simulink model "PMSM_MRAS"  (R2014b)
settings: Solver=ode23tb  StartTime=0.0  StopTime=0.4  FixedStep=5e-5  RelTol=1e-3
InitFcn:
  | L=8.5e-3;
  | R=2.875;
  | flux=0.175;
libraries: powerlib_extras x4, powerlib x4, simulink x1
settings Model: Creator=Paladin611  LastModifiedBy=Lei
settings DataIOCC: LimitDataPoints=off  SignalLoggingSaveFormat=ModelDataLogs
settings OptimizationCC: ExpressionDepthLimit=2147483647  InitFltsAndDblsToZero=on  EfficientMapNaN2IntZero=off
settings DebuggingCC: SaveWithParameterizedLinksMsg=none  UnderspecifiedInitializationDetection=Classic  MergeDetectMultiDrivingBlocksExec=none  SignalResolutionControl=TryResolveAllWithWarning  MultiTaskDSMMsg=warning  MultiTaskCondExecSysMsg=none  FcnCallInpInsideContextMsg=UseLocalSettings  StateNameClashWarn=warning
settings HardwareCC: TargetEndianess=LittleEndian  TargetHWDeviceType=MATLAB Host  ProdEqTarget=off
settings CodeAppCC: MaxIdLength=128
settings GRTTargetCC: CombineOutputUpdateFcns=off  GRTInterface=on

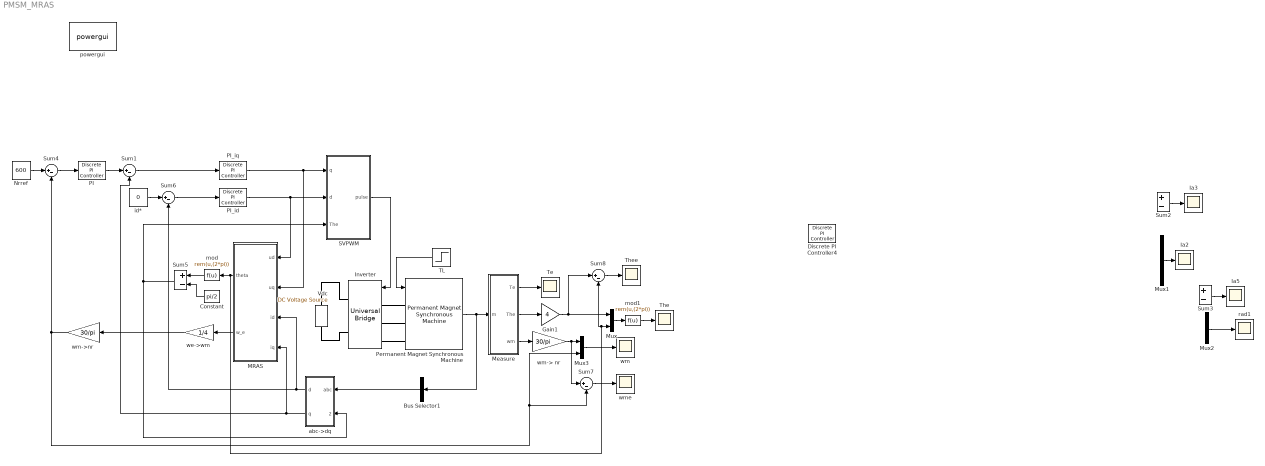
== system PMSM_MRAS ==
  Bus Selector1 : BusSelector  OutputSignals=Stator current is_a (A),Stator current is_b (A),Stator current is_c (A)  OutputAsBus=on
  Constant : Constant  Value=pi/2
  Discrete PI Controller4 : powerlib_extras/Discrete  Control Blocks/Discrete PI Controller  Kp=1*15  Ki=1000*4  Par_Limits=[1000 -1000]  Init=0  Ts=10e-6
  Gain1 : Gain  Gain=4
  Ia2 : Scope
      settings: TimeRange=0.1  YMin=-2  YMax=6.5  SaveName=ScopeData6
  Ia3 : Scope
      settings: TimeRange=0.1167052469135803  YMin=-6.5  YMax=2  SaveName=ScopeData7
  Ia5 : Scope
      settings: TimeRange=0.5  YMin=-100  YMax=150  SaveName=ScopeData11
  Inverter : powerlib/Power Electronics/Universal Bridge  Arms=3  SnubberResistance=1e5  SnubberCapacitance=inf  Device=IGBT / Diodes  Ron=1e-3  Lon=0  ForwardVoltages="[  0  0  ]"  ForwardVoltage=0  GTOparameters=[ 10e-6 , 20e-6 ]  IGBTparameters=[ 1e-6 , 2e-6 ]  Measurements=None  Measurements_2=None  converterType=Rectifier
  MRAS : Subsystem
  Measure : Subsystem
  Mux{,1..3} (4 alike) : Mux  Inputs=2
  Nrref : Constant  Value=600
  PI : powerlib_extras/Discrete  Control Blocks/Discrete PI Controller  Kp=0.068  Ki=17.1  Par_Limits=[100 -100]  Init=0  Ts=10e-6
  PI_id : powerlib_extras/Discrete  Control Blocks/Discrete PI Controller  Kp=L*2000  Ki=R*2000  Par_Limits=[300 -300]  Init=0  Ts=10e-6
  PI_iq : powerlib_extras/Discrete  Control Blocks/Discrete PI Controller  Kp=L*2000  Ki=R*2000  Par_Limits=[300 -300]  Init=0  Ts=10e-6
  Permanent Magnet Synchronous Machine : powerlib/Machines/Permanent Magnet Synchronous Machine  NbPhases=3  FluxDistribution=Sinusoidal  RotorType=Salient-pole  MechanicalLoad=Torque Tm  PresetModel=No  ShowDetailedParameters=on  MeasurementBus=off  Resistance=2.875  Inductance=8.5e-3  dqInductances=[8.5e-3 8.5e-3]  La=0.00085  MachineConstant=Flux linkage established by magnets (V.s)  Flux=0.175  VoltageCst=126.966  TorqueCst=1.05  Flat=120  Mechanical=[4.8e-6,0,4,0]  PolePairs=4  InitialConditions=[0,0, 0,0]  InitialConditions5ph=[0 0 0 0 0 0]  TsPowergui=0  TsBlock=-1  RefAngle=Aligned with phase A axis (original Park)
  SVPWM : Subsystem
  Sum{1,4,6..8} (5 alike) : Sum  Inputs=|+-
  Sum2 : Sum  Inputs=+-
  Sum3 : Sum  Inputs=+-
  Sum5 : Sum  Inputs=+-
  TL : Step  Time=0.3  After=0  SampleTime=0
  Te : Scope
      settings: TimeRange=0.01478751540608518  YMin=-7.5e-19  YMax=7.5e-19  SaveName=ScopeData10
  The : Scope
      settings: YMin=4.8  YMax=6.2  SaveName=The
  Thee : Scope
      settings: YMin=-0.4  YMax=0.05  SaveName=The1
  Vdc : powerlib/Electrical Sources/DC Voltage Source  Amplitude=311  Measurements=None
  abc->dq : Subsystem
  id* : Constant  Value=0
  mod : Fcn  Expr=rem(u,(2*pi))
  mod1 : Fcn  Expr=rem(u,(2*pi))
  powergui : powerlib/powergui  Priority=1  SimulationMode=Continuous  SolverType=Tustin  SampleTime=1e-6  frequency=60  SPID=off  DisableSnubberDevices=off  DisableRonSwitches=off  DisableVfSwitches=off  SwTol=0  DisplayEquations=off  Interpol=off  methode=off  Ts=0  frequencyindice=0  Pbase=100e6  ErrMax=1e-4  Iterations=50  UnitsV=kV  UnitsW=MW  FunctionMessages=off  echomessages=off  HookPort=off  EnableUseOfTLC=off  x0status=blocks  RestoreLinks=warning  ResistiveCurrentMeasurement=off  Frange=[0:2:500]  Ylog=off  Xlog=on  ShowGrid=off  save=off  variable=ZData  structure=0  ZoomFFT=off  StartTime=0.0  cycles=1  DisplayStyle=1  fundamental=60  FreqAxis=off  MaxFrequency=1000  frequencyindicesteady=1  RmsSteady=1  display=off
  rad1 : Scope
      settings: TimeRange=0.1  YMin=20  YMax=110  SaveName=ScopeData9
  we->wm : Gain  Gain=1/4
  wm : Scope
      settings: TimeRange=0.4  YMin=-200  YMax=1200  SaveName=wm
  wm-> nr : Gain  Gain=30/pi
  wm->nr : Gain  Gain=30/pi
  wme : Scope
      settings: TimeRange=0.4  YMin=-400  YMax=300  SaveName=wm1
  wires:
  Permanent Magnet Synchronous Machine/1 -> Measure/1(m), Bus Selector1/1
  Sum4/1 -> PI/1
  Sum1/1 -> PI_iq/1
  Sum6/1 -> PI_id/1
  Nrref/1 -> Sum4/1
  PI/1 -> Sum1/1
  Constant/1 -> Sum5/2
  ? -> Sum3/2, Mux2/2  "<Rotor speed wm (rad/s)>"
  ? -> Sum3/1, Mux2/1
  Mux1/1 -> Ia2/1
  Mux2/1 -> rad1/1
  Sum3/1 -> Ia5/1
  Sum2/1 -> Ia3/1
  ? -> Sum2/1
  ? -> Sum2/2
  ? -> Mux1/1
  ? -> Mux1/2
  id*/1 -> Sum6/1
  SVPWM/1(pulse) -> Inverter/1
  abc->dq/1(d) -> MRAS/3(id), Sum6/2
  abc->dq/2(q) -> Sum1/2, MRAS/4(iq)
  MRAS/2(w_e) -> we->wm/1
  we->wm/1 -> wm->nr/1
  Sum5/1 -> abc->dq/2(theta), SVPWM/3(The)
  PI_iq/1 -> MRAS/2(uq), SVPWM/1(q)
  PI_id/1 -> MRAS/1(ud), SVPWM/2(d)
  Measure/1(Te) -> Te/1
  Measure/2(The) -> Gain1/1
  Bus Selector1/1 -> abc->dq/1(abc)
  mod/1 -> Sum5/1
  Measure/3(wm) -> wm-> nr/1
  Mux3/1 -> wm/1
  wm->nr/1 -> Sum7/2, Mux3/2, Sum4/2
  wm-> nr/1 -> Sum7/1, Mux3/1
  Sum7/1 -> wme/1
  Sum8/1 -> Thee/1
  TL/1 -> Permanent Magnet Synchronous Machine/1
  Mux/1 -> mod1/1
  Gain1/1 -> Mux/1, Sum8/1
  MRAS/1(theta) -> Sum8/2, Mux/2, mod/1
  mod1/1 -> The/1
  connections:
  Vdc/LConn1 -- Inverter/RConn2
  Permanent Magnet Synchronous Machine/LConn1 -- Inverter/LConn1
  Permanent Magnet Synchronous Machine/LConn2 -- Inverter/LConn2
  Permanent Magnet Synchronous Machine/LConn3 -- Inverter/LConn3
  Vdc/RConn1 -- Inverter/RConn1

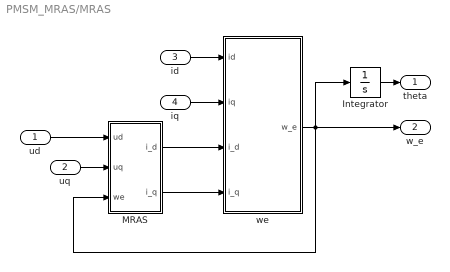
== system PMSM_MRAS/MRAS ==
  ud : Inport
  uq : Inport  Port=2
  id : Inport  Port=3
  iq : Inport  Port=4
  Integrator : Integrator
  MRAS : Subsystem
  we : Subsystem
  theta : Outport
  w_e : Outport  Port=2
  wires:
  ud/1 -> MRAS/1(ud)
  iq/1 -> we/2(iq)
  we/1(w_e) -> MRAS/3(we), w_e/1, Integrator/1
  uq/1 -> MRAS/2(uq)
  Integrator/1 -> theta/1
  MRAS/2(i_q) -> we/4(i_q)
  id/1 -> we/1(id)
  MRAS/1(i_d) -> we/3(i_d)

== system PMSM_MRAS/Measure ==
  m : Inport
  Bus Selector : BusSelector  OutputSignals=Electromagnetic torque Te (N*m),Rotor angle thetam (rad),Rotor speed wm (rad/s)
  Te : Outport
  The : Outport  Port=2
  wm : Outport  Port=3
  wires:
  Bus Selector/1 -> Te/1  "<Electromagnetic torque Te (N*m)>"
  Bus Selector/3 -> wm/1  "<Rotor speed wm (rad/s)>"
  Bus Selector/2 -> The/1  "<Rotor angle thetam (rad)>"
  m/1 -> Bus Selector/1

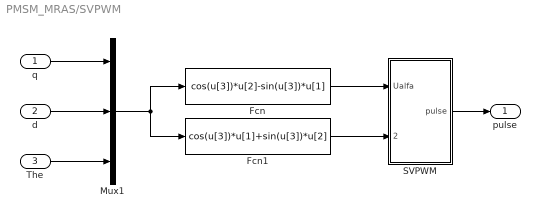
== system PMSM_MRAS/SVPWM ==
  q : Inport
  d : Inport  Port=2
  The : Inport  Port=3
  Fcn : Fcn  Expr=cos(u[3])*u[2]-sin(u[3])*u[1]
  Fcn1 : Fcn  Expr=cos(u[3])*u[1]+sin(u[3])*u[2]
  Mux1 : Mux  Inputs=3
  SVPWM : Subsystem  Tag=SVPWM  mask{F=10, Vdc=311}
      mask prompts: F "Chopping　Frequency(KHz)"; Vdc "DC Voltage(V)"
  pulse : Outport
  wires:
  The/1 -> Mux1/3
  Mux1/1 -> Fcn1/1, Fcn/1
  d/1 -> Mux1/2
  q/1 -> Mux1/1
  Fcn/1 -> SVPWM/1(Ualfa)
  Fcn1/1 -> SVPWM/2(Ubeta)
  SVPWM/1(pulse) -> pulse/1

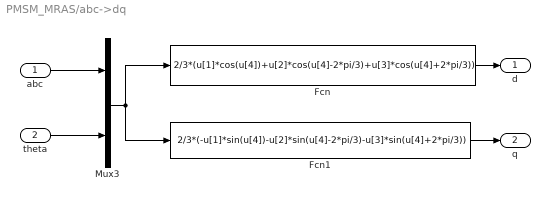
== system PMSM_MRAS/abc->dq ==
  abc : Inport
  theta : Inport  Port=2
  Fcn : Fcn  Expr=2/3*(u[1]*cos(u[4])+u[2]*cos(u[4]-2*pi/3)+u[3]*cos(u[4]+2*pi/3))
  Fcn1 : Fcn  Expr=2/3*(-u[1]*sin(u[4])-u[2]*sin(u[4]-2*pi/3)-u[3]*sin(u[4]+2*pi/3))
  Mux3 : Mux  Inputs=2
  d : Outport
  q : Outport  Port=2
  wires:
  Mux3/1 -> Fcn1/1, Fcn/1
  theta/1 -> Mux3/2
  Fcn/1 -> d/1
  Fcn1/1 -> q/1
  abc/1 -> Mux3/1

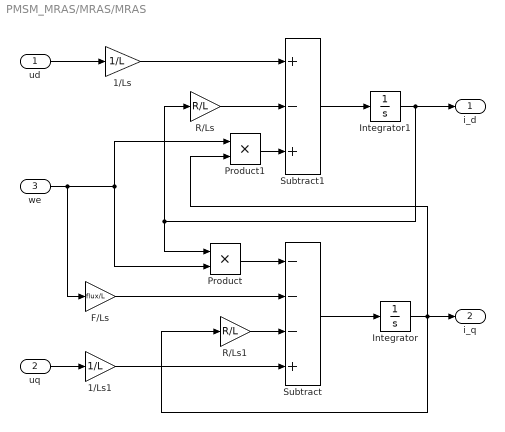
== system PMSM_MRAS/MRAS/MRAS ==
  ud : Inport
  uq : Inport  Port=2
  we : Inport  Port=3
  1/Ls : Gain  Gain=1/L
  1/Ls1 : Gain  Gain=1/L
  F/Ls : Gain  Gain=flux/L
  Integrator : Integrator
  Integrator1 : Integrator
  Product : Product  RndMeth=Zero
  Product1 : Product  RndMeth=Zero
  R/Ls : Gain  Gain=R/L
  R/Ls1 : Gain  Gain=R/L
  Subtract : Sum  Inputs=---+
  Subtract1 : Sum  Inputs=+-+
  i_d : Outport
  i_q : Outport  Port=2
  wires:
  1/Ls1/1 -> Subtract/4
  Subtract/1 -> Integrator/1
  Subtract1/1 -> Integrator1/1
  1/Ls/1 -> Subtract1/1
  Product1/1 -> Subtract1/3
  R/Ls/1 -> Subtract1/2
  Product/1 -> Subtract/1
  R/Ls1/1 -> Subtract/3
  uq/1 -> 1/Ls1/1
  we/1 -> F/Ls/1, Product/2, Product1/1
  F/Ls/1 -> Subtract/2
  Integrator1/1 -> R/Ls/1, Product/1, i_d/1
  ud/1 -> 1/Ls/1
  Integrator/1 -> R/Ls1/1, i_q/1, Product1/2

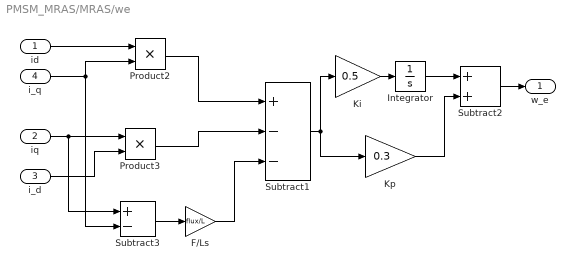
== system PMSM_MRAS/MRAS/we ==
  id : Inport
  iq : Inport  Port=2
  i_d : Inport  Port=3
  i_q : Inport  Port=4
  F/Ls : Gain  Gain=flux/L
  Integrator : Integrator
  Ki : Gain  Gain=0.5
  Kp : Gain  Gain=0.3
  Product2 : Product  RndMeth=Zero
  Product3 : Product  RndMeth=Zero
  Subtract1 : Sum  Inputs=+--
  Subtract2 : Sum
  Subtract3 : Sum  Inputs=+-
  w_e : Outport
  wires:
  id/1 -> Product2/1
  i_q/1 -> Subtract3/2, Product2/2
  iq/1 -> Subtract3/1, Product3/1
  i_d/1 -> Product3/2
  Subtract3/1 -> F/Ls/1
  F/Ls/1 -> Subtract1/3
  Subtract1/1 -> Ki/1, Kp/1
  Ki/1 -> Integrator/1
  Integrator/1 -> Subtract2/1
  Kp/1 -> Subtract2/2
  Product2/1 -> Subtract1/1
  Product3/1 -> Subtract1/2
  Subtract2/1 -> w_e/1

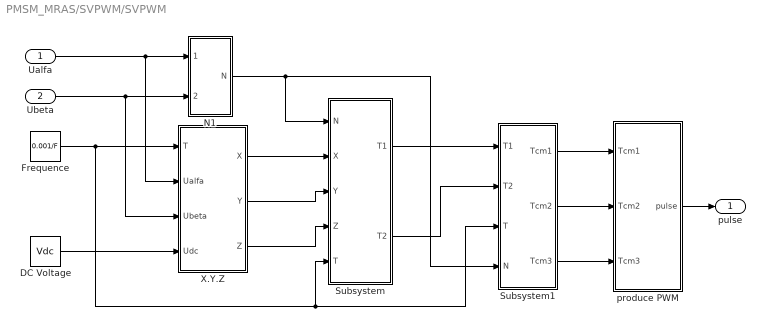
== system PMSM_MRAS/SVPWM/SVPWM ==
  Ualfa : Inport
  Ubeta : Inport  Port=2
  DC Voltage : Constant  Value=Vdc
  Frequence : Constant  Value=0.001/F
  N1 : Subsystem
  Subsystem : Subsystem
  Subsystem1 : Subsystem
  X.Y.Z : Subsystem
  produce PWM : Subsystem
  pulse : Outport
  wires:
  Ubeta/1 -> X.Y.Z/3(Ubeta), N1/2(Ubeta)
  Subsystem/2(T2) -> Subsystem1/2(T2)
  Subsystem/1(T1) -> Subsystem1/1(T1)
  Ualfa/1 -> N1/1(Ualfa), X.Y.Z/2(Ualfa)
  Subsystem1/3(Tcm3) -> produce PWM/3(Tcm3)
  Subsystem1/2(Tcm2) -> produce PWM/2(Tcm2)
  Subsystem1/1(Tcm1) -> produce PWM/1(Tcm1)
  X.Y.Z/3(Z) -> Subsystem/4(Z)
  X.Y.Z/2(Y) -> Subsystem/3(Y)
  X.Y.Z/1(X) -> Subsystem/2(X)
  N1/1(N) -> Subsystem1/4(N), Subsystem/1(N)
  DC Voltage/1 -> X.Y.Z/4(Udc)
  Frequence/1 -> Subsystem/5(T), Subsystem1/3(T), X.Y.Z/1(T)
  produce PWM/1(pulse) -> pulse/1

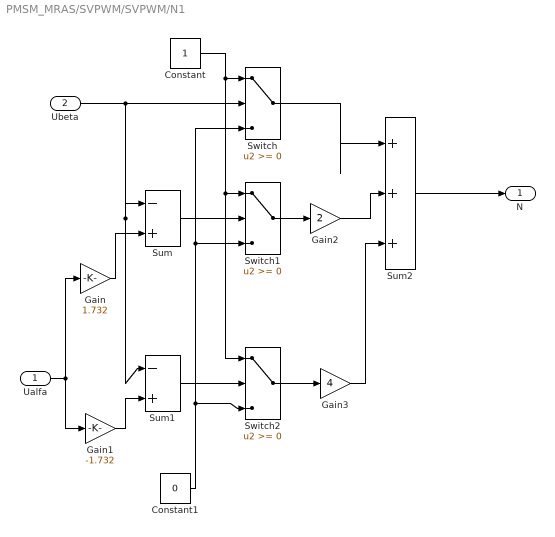
== system PMSM_MRAS/SVPWM/SVPWM/N1 ==
  Ualfa : Inport
  Ubeta : Inport  Port=2
  Constant : Constant
  Constant1 : Constant  Value=0
  Gain : Gain  Gain=1.732
  Gain1 : Gain  Gain=-1.732
  Gain2 : Gain  Gain=2
  Gain3 : Gain  Gain=4
  Sum : Sum  Inputs=|-+
  Sum1 : Sum  Inputs=|-+
  Sum2 : Sum  Inputs=|+++
  Switch : Switch
  Switch1 : Switch
  Switch2 : Switch
  N : Outport
  wires:
  Sum2/1 -> N/1
  Gain3/1 -> Sum2/3
  Switch/1 -> Sum2/1
  Gain2/1 -> Sum2/2
  Switch2/1 -> Gain3/1
  Switch1/1 -> Gain2/1
  Constant1/1 -> Switch2/3, Switch1/3, Switch/3
  Gain1/1 -> Sum1/2
  Sum1/1 -> Switch2/2
  Sum/1 -> Switch1/2
  Gain/1 -> Sum/2
  Ualfa/1 -> Gain/1, Gain1/1
  Constant/1 -> Switch1/1, Switch2/1, Switch/1
  Ubeta/1 -> Sum1/1, Sum/1, Switch/2

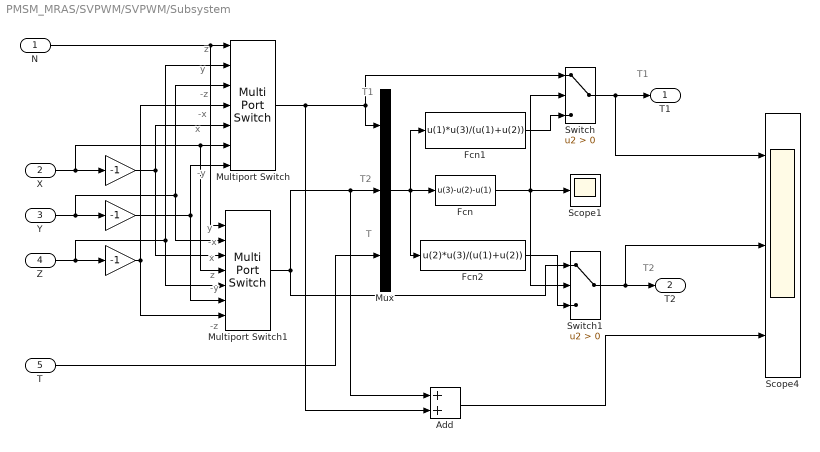
== system PMSM_MRAS/SVPWM/SVPWM/Subsystem ==
  note: T2
  note: T1
  note: T
  note: T2
  note: T1
  note: -z
  note: -y
  note: z
  note: x
  note: -x
  note: y
  note: -y
  note: x
  note: -x
  note: -z
  note: y
  note: z
  N : Inport
  X : Inport  Port=2
  Y : Inport  Port=3
  Z : Inport  Port=4
  T : Inport  Port=5
  " " : Gain  Gain=-1
  "  " : Gain  Gain=-1
  "    " : Gain  Gain=-1
  Add : Sum
  Fcn : Fcn  Expr=u(3)-u(2)-u(1)
  Fcn1 : Fcn  Expr=u(1)*u(3)/(u(1)+u(2))
  Fcn2 : Fcn  Expr=u(2)*u(3)/(u(1)+u(2))
  Multiport Switch : MultiPortSwitch  Inputs=6  DiagnosticForDefault=None
  Multiport Switch1 : MultiPortSwitch  Inputs=6  DiagnosticForDefault=None
  Mux : Mux  Inputs=3
  Scope1 : Scope
      settings: YMin=2  YMax=6  SaveName=ScopeData16
  Scope4 : Scope  NumInputPorts=3
      settings: TimeRange=0.5  YMin=-5e-05~-5e-05~0  YMax=9.999999999999999e-05~9.999999999999999e-05~0.008  SaveName=ScopeData4
  Switch : Switch  Criteria=u2 > Threshold
  Switch1 : Switch  Criteria=u2 > Threshold
  T1 : Outport
  T2 : Outport  Port=2
  wires:
  Add/1 -> Scope4/3
  Switch1/1 -> Scope4/2, T2/1
  Switch/1 -> Scope4/1, T1/1
  Fcn2/1 -> Switch1/3
  Fcn1/1 -> Switch/3
  Mux/1 -> Fcn2/1, Fcn1/1, Fcn/1
  T/1 -> Mux/3
  Multiport Switch/1 -> Add/2, Switch/1, Mux/1
  " "/1 -> Multiport Switch1/3, Multiport Switch/5
  "  "/1 -> Multiport Switch1/6, Multiport Switch/7
  "    "/1 -> Multiport Switch/4, Multiport Switch1/7
  Z/1 -> "    "/1, Multiport Switch/2, Multiport Switch1/5
  Y/1 -> "  "/1, Multiport Switch/3, Multiport Switch1/2
  X/1 -> " "/1, Multiport Switch/6, Multiport Switch1/4
  N/1 -> Multiport Switch/1, Multiport Switch1/1
  Fcn/1 -> Scope1/1, Switch1/2, Switch/2
  Multiport Switch1/1 -> Add/1, Mux/2, Switch1/1

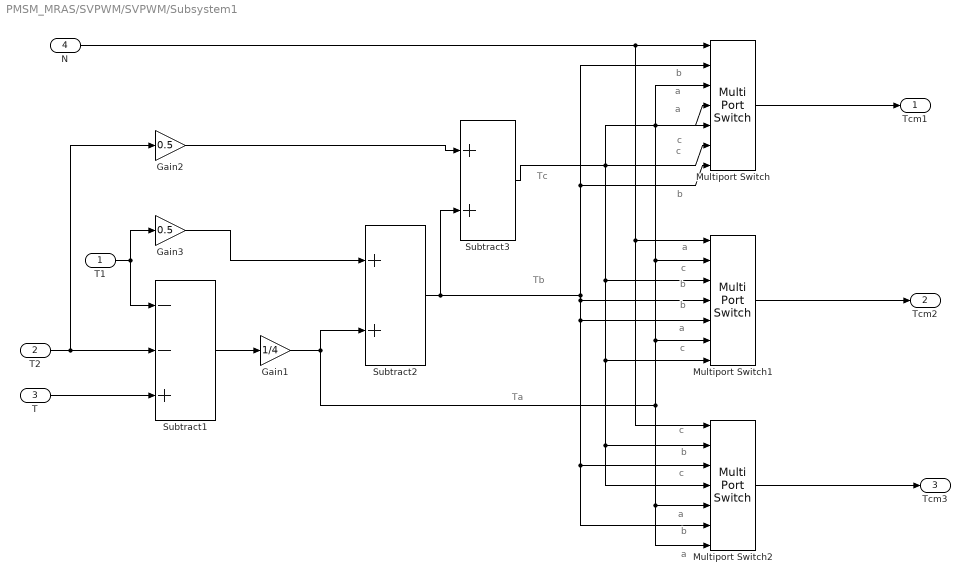
== system PMSM_MRAS/SVPWM/SVPWM/Subsystem1 ==
  note: a
  note: b
  note: a
  note: c
  note: b
  note: c
  note: c
  note: a
  note: b
  note: b
  note: c
  note: a
  note: b
  note: c
  note: c
  note: a
  note: a
  note: b
  note: Tc
  note: Tb
  note: Ta
  T1 : Inport
  T2 : Inport  Port=2
  T : Inport  Port=3
  N : Inport  Port=4
  Gain1 : Gain  Gain=1/4
  Gain2 : Gain  Gain=0.5
  Gain3 : Gain  Gain=0.5
  Multiport Switch : MultiPortSwitch  Inputs=6  DiagnosticForDefault=None
  Multiport Switch1 : MultiPortSwitch  Inputs=6  DiagnosticForDefault=None
  Multiport Switch2 : MultiPortSwitch  Inputs=6  DiagnosticForDefault=None
  Subtract1 : Sum  Inputs=--+
  Subtract2 : Sum
  Subtract3 : Sum
  Tcm1 : Outport
  Tcm2 : Outport  Port=2
  Tcm3 : Outport  Port=3
  wires:
  Subtract3/1 -> Multiport Switch2/4, Multiport Switch2/2, Multiport Switch1/7, Multiport Switch1/3, Multiport Switch/6, Multiport Switch/5
  N/1 -> Multiport Switch1/1, Multiport Switch2/1, Multiport Switch/1
  Gain2/1 -> Subtract3/1
  Subtract2/1 -> Multiport Switch2/6, Multiport Switch2/3, Multiport Switch1/5, Multiport Switch1/4, Multiport Switch/7, Multiport Switch/2, Subtract3/2
  Gain1/1 -> Subtract2/2, Multiport Switch1/6, Multiport Switch1/2, Multiport Switch/4, Multiport Switch/3, Multiport Switch2/7, Multiport Switch2/5
  Subtract1/1 -> Gain1/1
  Gain3/1 -> Subtract2/1
  T1/1 -> Subtract1/1, Gain3/1
  T/1 -> Subtract1/3
  T2/1 -> Subtract1/2, Gain2/1
  Multiport Switch/1 -> Tcm1/1
  Multiport Switch1/1 -> Tcm2/1
  Multiport Switch2/1 -> Tcm3/1

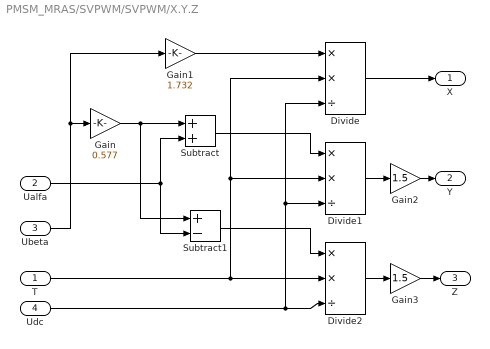
== system PMSM_MRAS/SVPWM/SVPWM/X.Y.Z ==
  T : Inport
  Ualfa : Inport  Port=2
  Ubeta : Inport  Port=3
  Udc : Inport  Port=4
  Divide : Product  Inputs=**/
  Divide1 : Product  Inputs=**/
  Divide2 : Product  Inputs=**/
  Gain : Gain  Gain=0.577
  Gain1 : Gain  Gain=1.732
  Gain2 : Gain  Gain=1.5
  Gain3 : Gain  Gain=1.5
  Subtract : Sum
  Subtract1 : Sum  Inputs=+-
  X : Outport
  Y : Outport  Port=2
  Z : Outport  Port=3
  wires:
  Ubeta/1 -> Gain/1, Gain1/1
  Gain3/1 -> Z/1
  Gain2/1 -> Y/1
  Divide2/1 -> Gain3/1
  Divide1/1 -> Gain2/1
  Divide/1 -> X/1
  Subtract1/1 -> Divide2/1
  Subtract/1 -> Divide1/1
  Ualfa/1 -> Subtract/2, Subtract1/2
  Udc/1 -> Divide/3, Divide1/3, Divide2/3
  T/1 -> Divide/2, Divide1/2, Divide2/2
  Gain1/1 -> Divide/1
  Gain/1 -> Subtract1/1, Subtract/1

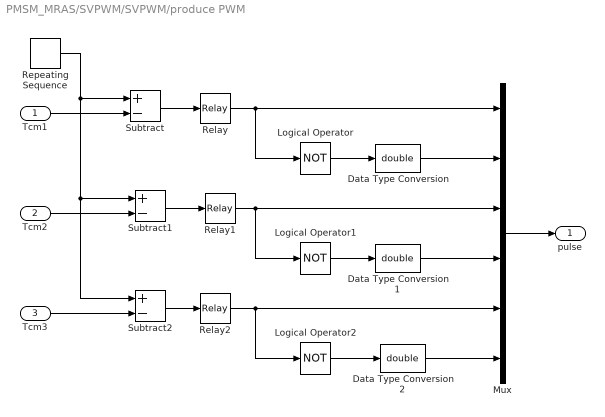
== system PMSM_MRAS/SVPWM/SVPWM/produce PWM ==
  Tcm1 : Inport
  Tcm2 : Inport  Port=2
  Tcm3 : Inport  Port=3
  Data Type Conversion : DataTypeConversion  OutDataTypeStr=double
  Data Type Conversion1 : DataTypeConversion  OutDataTypeStr=double
  Data Type Conversion2 : DataTypeConversion  OutDataTypeStr=double
  Logical Operator : Logic  Operator=NOT  AllPortsSameDT=off
  Logical Operator1 : Logic  Operator=NOT  AllPortsSameDT=off
  Logical Operator2 : Logic  Operator=NOT  AllPortsSameDT=off
  Mux : Mux  Inputs=6
  Relay : Relay
  Relay1 : Relay
  Relay2 : Relay
  Repeating Sequence : simulink/Sources/Repeating Sequence  rep_seq_t=[0 0.001/F 0.002/F]  rep_seq_y=[0 0.001/F 0]
  Subtract : Sum  Inputs=+-
  Subtract1 : Sum  Inputs=+-
  Subtract2 : Sum  Inputs=+-
  pulse : Outport
  wires:
  Data Type Conversion2/1 -> Mux/6
  Data Type Conversion1/1 -> Mux/4
  Data Type Conversion/1 -> Mux/2
  Mux/1 -> pulse/1
  Relay2/1 -> Mux/5, Logical Operator2/1
  Relay1/1 -> Mux/3, Logical Operator1/1
  Relay/1 -> Mux/1, Logical Operator/1
  Logical Operator/1 -> Data Type Conversion/1
  Logical Operator2/1 -> Data Type Conversion2/1
  Logical Operator1/1 -> Data Type Conversion1/1
  Tcm3/1 -> Subtract2/2
  Tcm2/1 -> Subtract1/2
  Tcm1/1 -> Subtract/2
  Repeating Sequence/1 -> Subtract1/1, Subtract2/1, Subtract/1
  Subtract2/1 -> Relay2/1
  Subtract1/1 -> Relay1/1
  Subtract/1 -> Relay/1
